simulink model "ex2_Q3"  (R2024a)
settings: Solver=FixedStepDiscrete  StartTime=0.0  StopTime=10.0  FixedStep=0.0001  RelTol=1e-3
settings Model: Creator=erfuu  LastModifiedBy=erfuu

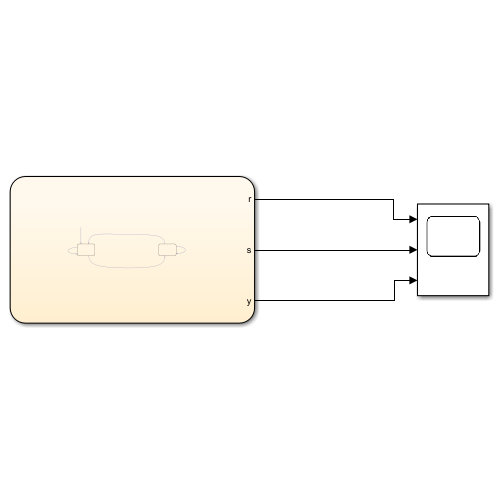
[thumbnail: Simulink's stored preview of the top-level diagram]
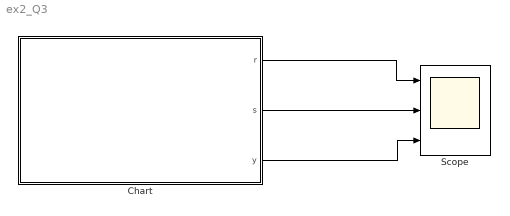
== system ex2_Q3 ==
  Chart : Stateflow chart  TreatAsAtomicUnit=on
  Scope : Scope  NumInputPorts=3
  wires:
  Chart/1(r) -> Scope/1
  Chart/2(s) -> Scope/2
  Chart/3(y) -> Scope/3

== stateflow chart ex2_Q3/Chart ==
  state one
  state two
  (default) -> one : {s = 0; r = 0; y = 0}
  two -> one [order 1] : [r > 2  - interval]{y = s; r = 0;}
  two -> two [order 2] : [r < 2]{s = s + (1 * interval); r  = r + (1 * interval);}
  one -> one [order 2] : [r < 1]{s = s + (1 * interval); r  = r + (1 * interval);}
  one -> two [order 1] : [r > 1 - interval]{y = s; r = 0}
  data: r output; s output; interval constant double =0.0001; y output
